simulink model "Parking_NMPC_MultiStage_Controller"  (R2024b)
settings: configuration reference "vehicle_nl_controller_config" (kept outside this file)
undefined symbols (not defined in the file or in its folder): convert_theta_to_q, nl_vehicle_MPC_lib, refNum, TimeStep, u0, weight_dmv, weight_mv, weight_x, wheel_base
libraries: mpclib x1
settings Model: DataDictionary=sim_data_vehicle_nl.sldd  Creator=tshintai  LastModifiedBy=tshintai
settings ConfigSetRef: SourceName=vehicle_nl_controller_config

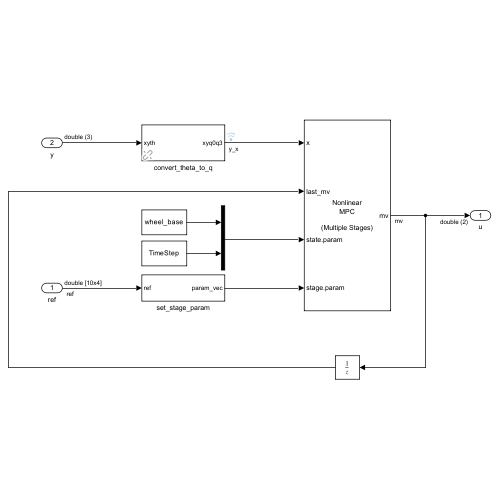
[thumbnail: Simulink's stored preview of the top-level diagram]
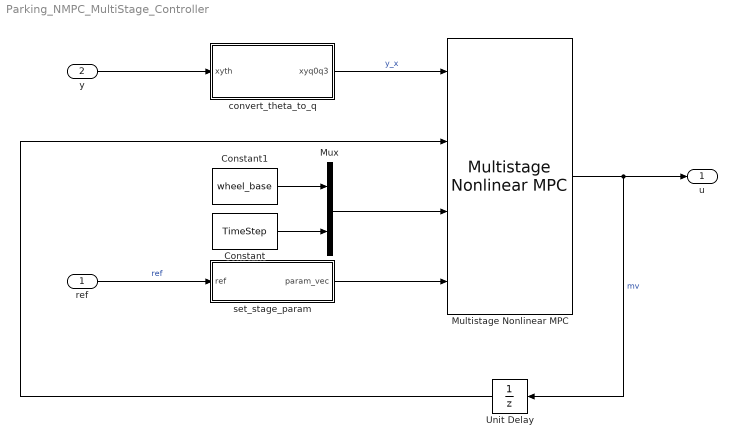
== system Parking_NMPC_MultiStage_Controller ==
  ref : Inport  OutDataTypeStr=double  PortDimensions=[refNum, 4]
  y : Inport  Port=2  OutDataTypeStr=double  PortDimensions=3
  Constant : Constant  Value=TimeStep
  Constant1 : Constant  Value=wheel_base
  Multistage Nonlinear MPC : mpclib/Multistage Nonlinear MPC  SCDEnableBlockLinearizationSpecification=on  nlmpcobj=nlMPCObj  UseObjectTs=on  TsControl=-1  UseMEX=off  mexname=''  md_enabled=off  stateparam_enabled=on  stageparam_enabled=on  cost_enabled=off  mvseq_enabled=off  stateseq_enabled=off  slack_enabled=off  status_enabled=off  mv_min=off  mv_max=off  mvrate_min=off  mvrate_max=off  state_min=off  state_max=off  terminal_state=off  nlp_initialize=off
  Mux : Mux  Inputs=2
  Unit Delay : UnitDelay  InitialCondition=u0  SampleTime=-1  HasFrameUpgradeWarning=on
  convert_theta_to_q : Subsystem  AncestorBlock=nl_vehicle_MPC_lib/convert_theta_to_q
  set_stage_param : Subsystem
  u : Outport  OutDataTypeStr=double  PortDimensions=2
  wires:
  Multistage Nonlinear MPC/1 -> u/1, Unit Delay/1  "mv"
  Unit Delay/1 -> Multistage Nonlinear MPC/2
  y/1 -> convert_theta_to_q/1(xyth)
  Constant/1 -> Mux/2
  Constant1/1 -> Mux/1
  convert_theta_to_q/1(xyq0q3) -> Multistage Nonlinear MPC/1  "y_x"
  ref/1 -> set_stage_param/1(ref)  "ref"
  Mux/1 -> Multistage Nonlinear MPC/3
  set_stage_param/1(param_vec) -> Multistage Nonlinear MPC/4

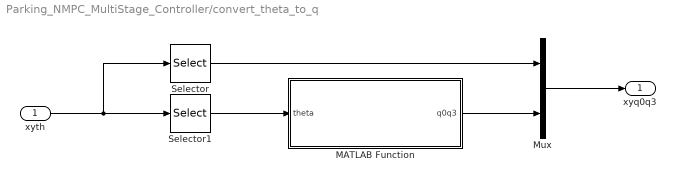
== system Parking_NMPC_MultiStage_Controller/convert_theta_to_q ==
  xyth : Inport
  MATLAB Function : MATLAB Function  TreatAsAtomicUnit=on
  Mux : Mux  Inputs=2
  Selector : Selector  InputPortWidth=3  IndexOptions=Index vector (dialog)  Indices=[1 2]  OutputSizes=1
  Selector1 : Selector  InputPortWidth=3  IndexOptions=Index vector (dialog)  Indices=[3]  OutputSizes=1
  xyq0q3 : Outport
  wires:
  Selector/1 -> Mux/1
  Mux/1 -> xyq0q3/1
  xyth/1 -> Selector/1, Selector1/1
  Selector1/1 -> MATLAB Function/1(theta)
  MATLAB Function/1(q0q3) -> Mux/2

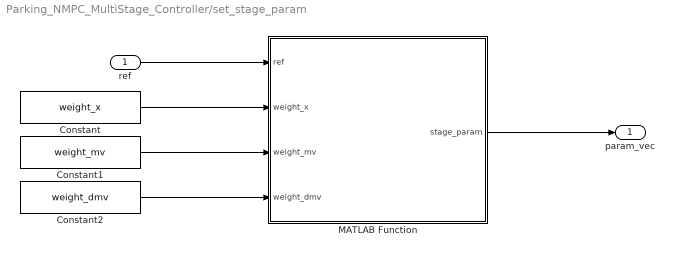
== system Parking_NMPC_MultiStage_Controller/set_stage_param ==
  ref : Inport
  Constant : Constant  Value=weight_x  VectorParams1D=off
  Constant1 : Constant  Value=weight_mv  VectorParams1D=off
  Constant2 : Constant  Value=weight_dmv  VectorParams1D=off
  MATLAB Function : MATLAB Function  TreatAsAtomicUnit=on
  param_vec : Outport
  wires:
  ref/1 -> MATLAB Function/1(ref)
  MATLAB Function/1(stage_param) -> param_vec/1
  Constant/1 -> MATLAB Function/2(weight_x)
  Constant1/1 -> MATLAB Function/3(weight_mv)
  Constant2/1 -> MATLAB Function/4(weight_dmv)

== matlab function Parking_NMPC_MultiStage_Controller/convert_theta_to_q/MATLAB Function ==
  data: theta input; q0q3 output
function q0q3 = theta_to_q0q3_no_outlier(theta)

persistent initial_flag;
if isempty(initial_flag)
    initial_flag = false;
end
persistent q0q3_pre;
if isempty(q0q3_pre)
    q0q3_pre = zeros(2, 1, 'like', theta);
end

THETA = 0.5 * theta;
q0q3 = [cos(THETA); sin(THETA)];

if (~initial_flag)
    q0q3_pre = q0q3;
    initial_flag = true;
else
    diff = sum(abs(q0q3 - q0q3_pre));
        
    if (diff > 0.5)
        THETA_2 = 0.5 * (theta + 2 * pi);
        q0q3 = [cos(THETA_2); sin(THETA_2)];
        q0q3_pre = q0q3;
    else
        q0q3_pre = q0q3;
    end

end

end

== matlab function Parking_NMPC_MultiStage_Controller/set_stage_param/MATLAB Function ==
  data: ref input; stage_param output; weight_x input; weight_mv input; weight_dmv input
function stage_param = set_stage_param(ref, weight_x, weight_mv, weight_dmv)

% 参照軌道の行列に重みを接続する。
weight_vec = [weight_x, weight_mv, weight_dmv];
MAT = [ref, repmat(weight_vec, size(ref, 1), 1)];

% 行列をベクトルに変換する。
stage_param = reshape(MAT', [], 1);

end
